simulink model "case_study_sync_buck_boost"  (R2017b)
settings: Solver=ode1  StartTime=0.0  StopTime=1e-3  FixedStep=10e-9  RelTol=1e-3
PostLoadFcn:
  | , if any(exist('dsrtsu_mdlpostloadfcn', 'file') == [2, 3, 6]), try dsrtsu_mdlpostloadfcn('Execute', bdroot); catch fprintf('Error in PostLoadFcn (dsrtsu_mdlpostloadfcn) for model "%s":\n %s\n', bdroot, lasterr); end, end,
InitFcn:
  | run('init_synchronous_buck_boost.m');
values from neighbouring files (symbols this model uses):
  Vin = 5    [init_synchronous_buck_boost.m]
  Vmax = 10    [init_synchronous_buck_boost.m]
  Vref = 2.5    [init_synchronous_buck_boost.m]
libraries: simulink x1
Description:
  | Standard RTI1005 template.
  | Supported MATLAB version:  R2017b.
settings Model: Tag=RTI1005  DSRTSU_INTERNAL_RTI_VER=540  DSRTSU_INTERNAL_RTI_TYPE=rti1005  RTICANMMDATA=struct('GeneralSetupData',struct('modelroot','C:\Projects\Simulink\PE_1\w2','generalsettings',struct('filesettings',struct('destfolder',struct('Name','RTICANMM_FILES','Check',1),'buildfolder',struct('Name','.','Check',1),'AbsDestfolder',struct('Name','C:\Projects\Simulink\PE_1\w2\RTICANMM_FILES'),'AbsBuildfolder',struct('Name','C:\Projects\Simulink\PE_1\w2'))),'options',struct('addpaths',1,'rmpaths',1,'addtrcexclusion',logical(1),'cannavigator',struct('checkmonitoring',0),'show_usrtrc',0,'use_usrtrc',0),'advanced',struct('options',ones(1,100)),'MPSetup',{{}},'RTI',struct('Type','RTI1005','Ver','7.12','Date','02-May-2019'),'modelname','case_study_sync_buck_boost','block','case_study_sync_buck_boost'))  DSRTSU_INTERNAL_RTIFPGA=130  Creator=CA72672  LastModifiedBy=CA72672
settings OptimizationCC: BlockReduction=off  OptimizeBlockIOStorage=off  BufferReuse=off  GlobalBufferReuse=off  ExpressionFolding=off  LocalBlockOutputs=off
settings HardwareCC: ProdBitPerPointer=32  ProdBitPerSizeT=32  ProdBitPerPtrDiffT=32  ProdLargestAtomicInteger=Integer  ProdEndianess=BigEndian  ProdWordSize=32  ProdHWDeviceType=Custom Processor->Custom  TargetIntDivRoundTo=Zero  TargetEndianess=BigEndian  TargetHWDeviceType=Custom Processor->Custom
settings SFSimCC: MATLABDynamicMemAlloc=off
settings RTWCC: SystemTargetFile=rti1005.tlc  MakeCommand=make_rti  TemplateMakefile=rti1005.tmf  Description=dSPACE DS1005 Hardware Platform
settings CodeAppCC: StateflowObjectComments=on
settings STFCustomTargetCC: ParMdlRefBuildCompliant=on  MatFileLogging=on  GRTInterface=off  SystemTargetFile=rti1005.tlc
settings GRTTargetCC: TargetLangStandard=C89/C90 (ANSI)  CompOptLevelCompliant=off  ConcurrentExecutionCompliant=off  CombineOutputUpdateFcns=off  CPPClassGenCompliant=off  UseToolchainInfoCompliant=off
settings ConfigComp: CovMetricSettings=dswe

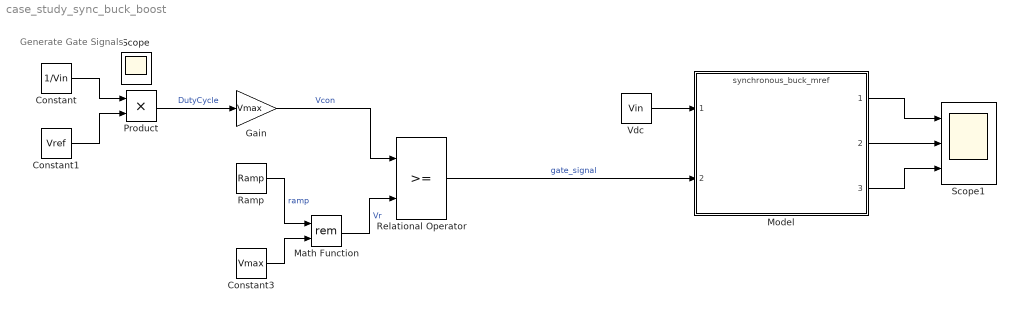
== system case_study_sync_buck_boost ==
  note: Generate Gate Signals
  Constant : Constant  Value=1/Vin
  Constant1 : Constant  Value=Vref
  Constant3 : Constant  Value=Vmax
  Gain : Gain  Gain=Vmax
  Math Function : Math  Operator=rem  SaturateOnIntegerOverflow=on
  Model : ModelReference  ModelNameDialog=synchronous_buck_mref.slx  SimulationMode=Normal  ModelReferenceVersion=1.1
  Product : Product
  Ramp : simulink/Sources/Ramp  slope=Vmax/Tsw  start=0  X0=0
  Relational Operator : RelationalOperator  OutDataTypeStr=boolean  RndMeth=Simplest
  Scope1 : Scope  NumInputPorts=3
  Vdc : Constant  Value=Vin
  Scope : Scope
  wires:
  Constant1/1 -> Product/2
  Constant/1 -> Product/1
  Product/1 -> Gain/1  "DutyCycle"
  Gain/1 -> Relational Operator/1  "Vcon"
  Ramp/1 -> Math Function/1  "ramp"
  Constant3/1 -> Math Function/2
  Math Function/1 -> Relational Operator/2  "Vr"
  Relational Operator/1 -> Model/2  "gate_signal"
  Vdc/1 -> Model/1
  Model/2 -> Scope1/2
  Model/1 -> Scope1/1
  Model/3 -> Scope1/3
